simulink model "complete_controller_organized"  (R2023a)
settings: Solver=FixedStepAuto  StartTime=0.0  StopTime=inf  FixedStep=0.01  RelTol=1e-3
model workspace (MAT data in the model file):
  SL_ROS_VariableLengthArrays_MaxSizes.CommonInfo.ArrayTruncateAction = 'EmitWarning'
  SL_ROS_VariableLengthArrays_MaxSizes.MsgTypeMap = containers.Map
  SL_ROS_VariableLengthArrays_MaxSizes.MsgTypeMap.serialization.keys = {'diagnostic_msgs/DiagnosticArray', 'diagnostic_msgs/DiagnosticStatus', 'std_msgs/Float32MultiArray', 'std_msgs/Int32MultiArray'}
  SL_ROS_VariableLengthArrays_MaxSizes.MsgTypeMap.serialization.values{1}.PropertyName = 'status'
  SL_ROS_VariableLengthArrays_MaxSizes.MsgTypeMap.serialization.values{1}.DataType = 'diagnostic_msgs/DiagnosticStatus'
  SL_ROS_VariableLengthArrays_MaxSizes.MsgTypeMap.serialization.values{1}.MaxLength = 2
  SL_ROS_VariableLengthArrays_MaxSizes.MsgTypeMap.serialization.values{2}(1).PropertyName = 'hardware_id'
  SL_ROS_VariableLengthArrays_MaxSizes.MsgTypeMap.serialization.values{2}(1).DataType = 'uint8'
  SL_ROS_VariableLengthArrays_MaxSizes.MsgTypeMap.serialization.values{2}(1).MaxLength = 128
  SL_ROS_VariableLengthArrays_MaxSizes.MsgTypeMap.serialization.values{2}(2).PropertyName = 'message'
  SL_ROS_VariableLengthArrays_MaxSizes.MsgTypeMap.serialization.values{2}(2).DataType = 'uint8'
  SL_ROS_VariableLengthArrays_MaxSizes.MsgTypeMap.serialization.values{2}(2).MaxLength = 128
  SL_ROS_VariableLengthArrays_MaxSizes.MsgTypeMap.serialization.values{2}(3).PropertyName = 'name'
  SL_ROS_VariableLengthArrays_MaxSizes.MsgTypeMap.serialization.values{2}(3).DataType = 'uint8'
  SL_ROS_VariableLengthArrays_MaxSizes.MsgTypeMap.serialization.values{2}(3).MaxLength = 128
  SL_ROS_VariableLengthArrays_MaxSizes.MsgTypeMap.serialization.values{2}(4).PropertyName = 'values'
  SL_ROS_VariableLengthArrays_MaxSizes.MsgTypeMap.serialization.values{2}(4).DataType = 'diagnostic_msgs/KeyValue'
  SL_ROS_VariableLengthArrays_MaxSizes.MsgTypeMap.serialization.values{2}(4).MaxLength = 8
  SL_ROS_VariableLengthArrays_MaxSizes.MsgTypeMap.serialization.values{3}.PropertyName = 'data'
  SL_ROS_VariableLengthArrays_MaxSizes.MsgTypeMap.serialization.values{3}.DataType = 'single'
  SL_ROS_VariableLengthArrays_MaxSizes.MsgTypeMap.serialization.values{3}.MaxLength = 8
  SL_ROS_VariableLengthArrays_MaxSizes.MsgTypeMap.serialization.values{4}.PropertyName = 'data'
  SL_ROS_VariableLengthArrays_MaxSizes.MsgTypeMap.serialization.values{4}.DataType = 'int32'
  SL_ROS_VariableLengthArrays_MaxSizes.MsgTypeMap.serialization.values{4}.MaxLength = 8
  SL_ROS_VariableLengthArrays_MaxSizes.MsgTypeMap.serialization.uniformity = 0
  SL_ROS_VariableLengthArrays_MaxSizes.MsgTypeMap.serialization.keyType = 'char'
  SL_ROS_VariableLengthArrays_MaxSizes.MsgTypeMap.serialization.valueType = 'any'
undefined symbols (not defined in the file): adjusted_FF, angular, Btrigger_boost, DAapply_nudges, DAdesired_pose, DAff_body_force, DAsolver_weights, Djoy_R_X, Dreverse_throttle, Dthrottle, Iangular_mode, Ilinear_mode, linear, reading, standard_variance, status, true_trust
libraries: ros2lib x78
(part 1 of 2)
settings Model: Creator=john  LastModifiedBy=john
settings OptimizationCC: GainParamInheritBuiltInType=on  UseFloatMulNetSlope=on  EnhancedBackFolding=on  PassReuseOutputArgsAs=Individual arguments  ZeroExternalMemoryAtStartup=off  ZeroInternalMemoryAtStartup=off  MaxStackSize=64  OptimizeBlockOrder=speed  DifferentSizesBufferReuse=on  OptimizationCustomize=off  EfficientTunableParamExpr=on
settings DebuggingCC: ParameterTunabilityLossMsg=error  UnderSpecifiedDimensionMsg=warning
settings HardwareCC: ProdBitPerLong=64  ProdHWDeviceType=Intel->x86-64 (Linux 64)
settings SFSimCC: SimUserSources=complete_system/send_thruster_cmd_canbus.c  SimTargetLang=C++
settings RTWCC: Description=Embedded Coder  SystemTargetFile=ert.tlc  HardwareBoard=Robot Operating System 2 (ROS 2)  TLCOptions="-aInlineSetEventsForThisBaseRateFcn=TLC_FALSE -aSuppressMultiTaskScheduler=TLC_FALSE  -aRateBasedStepFcn=0"  TemplateMakefile=ert_default_tmf  Toolchain=Colcon Tools  TargetLang=C++
settings CodeAppCC: ForceParamTrailComments=on  IgnoreCustomStorageClasses=off  OperatorAnnotations=on  SimulinkDataObjDesc=on  SFDataObjDesc=on  InsertBlockDesc=on
settings ERTTargetCC: CodeInterfacePackaging=C++ class  RootIOFormat=Structure reference

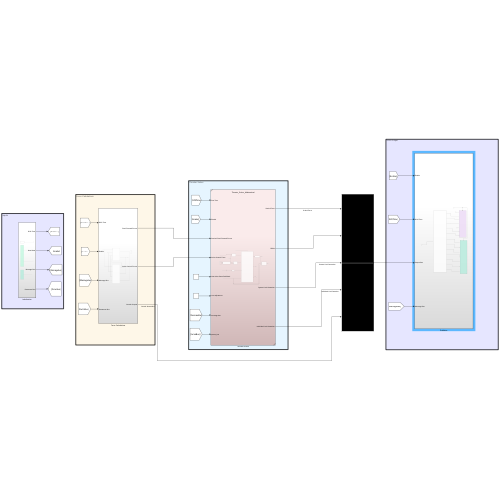
[thumbnail: Simulink's stored preview of the top-level diagram]
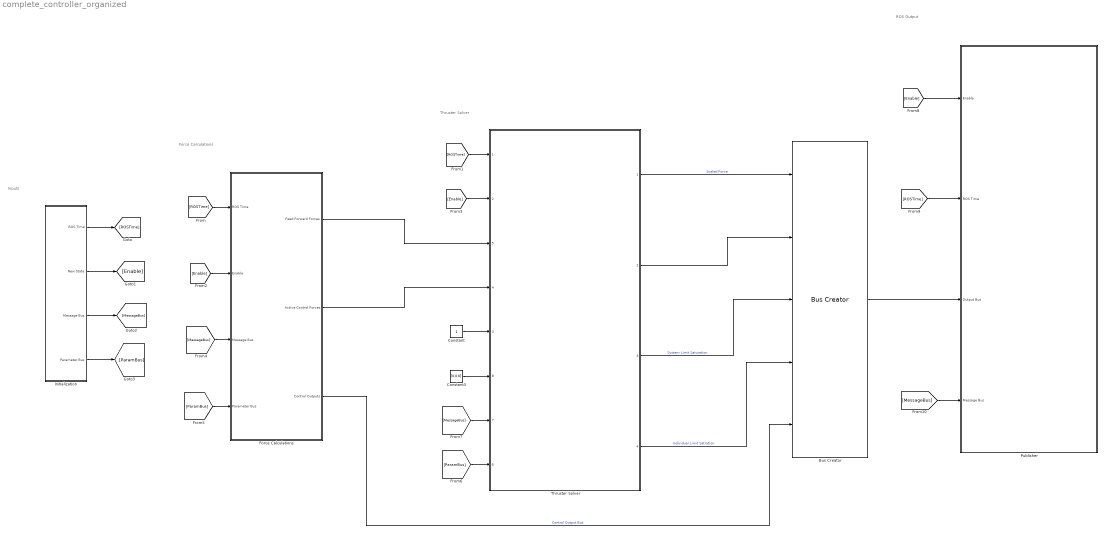
== system complete_controller_organized ==
  note: ROS Output
  note: Thruster Solver
  note: Force Calculations
  note: Inputs
  Bus Creator : BusCreator  Inputs=5
  Constant : Constant
  Constant3 : Constant  Value=[0,0,0]
  Force Calculations : Subsystem
  Initialization : Subsystem
  Publisher : Subsystem
  Thruster Solver : Subsystem  ReferencedSubsystem=Thruster_Solver_Mathmatical
      settings: PortSchema="{\"entries\":[{\"content\":{\"sides\":[{\"content\":{\"connectorIds\":[\"In1\",\"In2\",\"In5\",\"In4\",\"In3\",\"In8\",\"In7\",\"In6\"]},\"type\":\"ConnectorPlacement.EquallySpacedRectSide\",\"uuid\":\"7443c28d-8cee-4065-b63f-8039eaddf426\"},{\"content\":{\"connectorIds\":[\"Out1\",\"Out2\",\"Out3\",\"Out4\"],\"side\":\"RIGHT\"},\"type\":\"ConnectorPlacement.EquallySpacedRectSide\",\"uuid\":\"625b2eba-64d9-4ade-9893-8e78eb613954\"},{\"content\":{\"side\":\"TOP\"},\"type\":\"ConnectorPlacement.EquallySpacedRectSide\",\"uuid\":\"e2df6dfc-d16d-465d-896d-535154799a49\"}]},\"type\":\"ConnectorPlacement.EquallySpacedConnector\",\"uuid\":\"d998c598-ebfe-49fc-a537-223cf8fafed3\"}],\"packageUris\":[\"http://schema.mathworks.com/mf0/Connector/R2020b\"],\"version\":\"1.0\"}"
  wires:
  Force Calculations/1(Feed Forward Forces) -> Thruster Solver/5
  Force Calculations/2(Active Control Forces) -> Thruster Solver/4
  Constant/1 -> Thruster Solver/3
  Constant3/1 -> Thruster Solver/8
  Initialization/1(ROS Time) -> [ROSTime]
  [ROSTime] -> Force Calculations/1(ROS Time)
  [ROSTime] -> Thruster Solver/1
  Initialization/2(New State) -> [Enable]
  [Enable] -> Force Calculations/2(Enable)
  [Enable] -> Thruster Solver/2
  Initialization/3(Message Bus) -> [MessageBus]
  [MessageBus] -> Force Calculations/3(Message Bus)
  Initialization/4(Parameter Bus) -> [ParamBus]
  [ParamBus] -> Force Calculations/4(Parameter Bus)
  [ParamBus] -> Thruster Solver/6
  [MessageBus] -> Thruster Solver/7
  Thruster Solver/1 -> Bus Creator/1  "Scaled Force"
  Thruster Solver/2 -> Bus Creator/2
  Thruster Solver/3 -> Bus Creator/3  "System Limit Saturation"
  Thruster Solver/4 -> Bus Creator/4  "Individual Limit Satration"
  Force Calculations/3(Control Outputs) -> Bus Creator/5  "Control Output Bus"
  Bus Creator/1 -> Publisher/3(Output Bus)
  [Enable] -> Publisher/1(Enable)
  [ROSTime] -> Publisher/2(ROS Time)
  [MessageBus] -> Publisher/4(Message Bus)

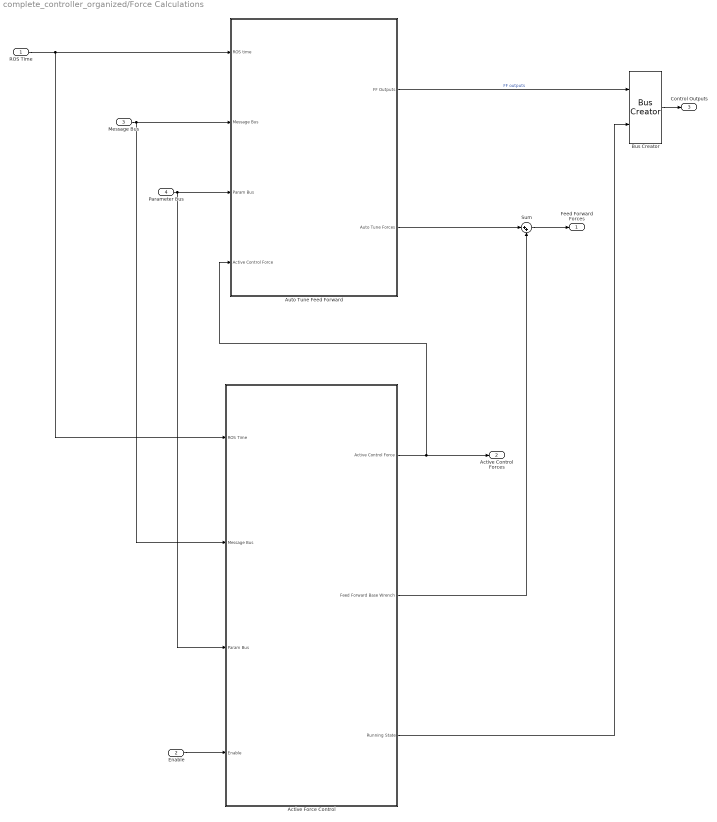
== system complete_controller_organized/Force Calculations ==
  ROS Time : Inport
  Enable : Inport  Port=2
  Message Bus : Inport  Port=3
  Parameter Bus : Inport  Port=4
  Active Force Control : Subsystem
  Auto Tune Feed Forward : Subsystem
  Bus Creator : BusCreator  Inputs=2
  Sum : Sum  Inputs=|++
  Feed Forward Forces : Outport
  Active Control Forces : Outport  Port=2
  Control Outputs : Outport  Port=3
  wires:
  Active Force Control/1(Active Control Force) -> Active Control Forces/1, Auto Tune Feed Forward/4(Active Control Force)
  Sum/1 -> Feed Forward Forces/1
  Auto Tune Feed Forward/2(Auto Tune Forces) -> Sum/1
  Active Force Control/2(Feed Forward Base Wrench) -> Sum/2
  Auto Tune Feed Forward/1(FF Outputs) -> Bus Creator/1  "FF outputs"
  Active Force Control/3(Running State) -> Bus Creator/2
  Bus Creator/1 -> Control Outputs/1
  ROS Time/1 -> Active Force Control/1(ROS Time), Auto Tune Feed Forward/1(ROS time)
  Enable/1 -> Active Force Control/4(Enable)
  Message Bus/1 -> Auto Tune Feed Forward/2(Message Bus), Active Force Control/2(Message Bus)
  Parameter Bus/1 -> Auto Tune Feed Forward/3(Param Bus), Active Force Control/3(Param Bus)

== system complete_controller_organized/Initialization ==
  Current Time : ros2lib/Current Time  OutputFormat=double  SampleTime=-1  ModelName=complete_controller_organized
  Subsystem : Subsystem
  Subsystem1 : Subsystem
  ROS Time : Outport
  New State : Outport  Port=2
  Message Bus : Outport  Port=3
  Parameter Bus : Outport  Port=4
  wires:
  Current Time/1 -> ROS Time/1
  Subsystem1/1(New State) -> New State/1
  Subsystem1/2(Message Bus) -> Message Bus/1
  Subsystem/1(param_bus) -> Parameter Bus/1  "param bus"

== system complete_controller_organized/Publisher ==
  Enable : Inport
  ROS Time : Inport  Port=2
  Output Bus : Inport  Port=3
  Message Bus : Inport  Port=4
  Bus Selector : BusSelector  OutputSignals=RPMs,System Limit Saturation,Individual Limit Satration,Control Output Bus.FF outputs.status,Control Output Bus.FF outputs.reading,Scaled Force,RPMs,Control Output Bus.running_state,Control Output Bus.FF outputs.adjusted_FF,Control Output Bus.FF outputs.reading,Control Output Bus.FF outputs.standard_variance,Control Output Bus.FF outputs.true_trust
  Publish System : Subsystem  ReferencedSubsystem=Publish_Control_System_Out
  Subsystem Reference3 : Subsystem  ReferencedSubsystem=Diagnostic_Reporter
  wires:
  Enable/1 -> Publish System/Enable, Subsystem Reference3/Enable
  Output Bus/1 -> Bus Selector/1
  ROS Time/1 -> Subsystem Reference3/1
  Message Bus/1 -> Subsystem Reference3/5
  Bus Selector/1 -> Subsystem Reference3/2  "<RPMs>"
  Bus Selector/2 -> Subsystem Reference3/3  "<System Limit Saturation>"
  Bus Selector/3 -> Subsystem Reference3/4  "<Individual Limit Satration>"
  Bus Selector/4 -> Subsystem Reference3/6  "<status>"
  Bus Selector/5 -> Subsystem Reference3/7  "<reading>"
  Bus Selector/6 -> Publish System/1  "<Scaled Force>"
  Bus Selector/7 -> Publish System/2  "<RPMs>"
  Bus Selector/8 -> Publish System/3  "<running_state>"
  Bus Selector/9 -> Publish System/4  "<adjusted_FF>"
  Bus Selector/10 -> Publish System/5  "<reading>"
  Bus Selector/11 -> Publish System/6  "<standard_variance>"
  Bus Selector/12 -> Publish System/7  "<true_trust>"

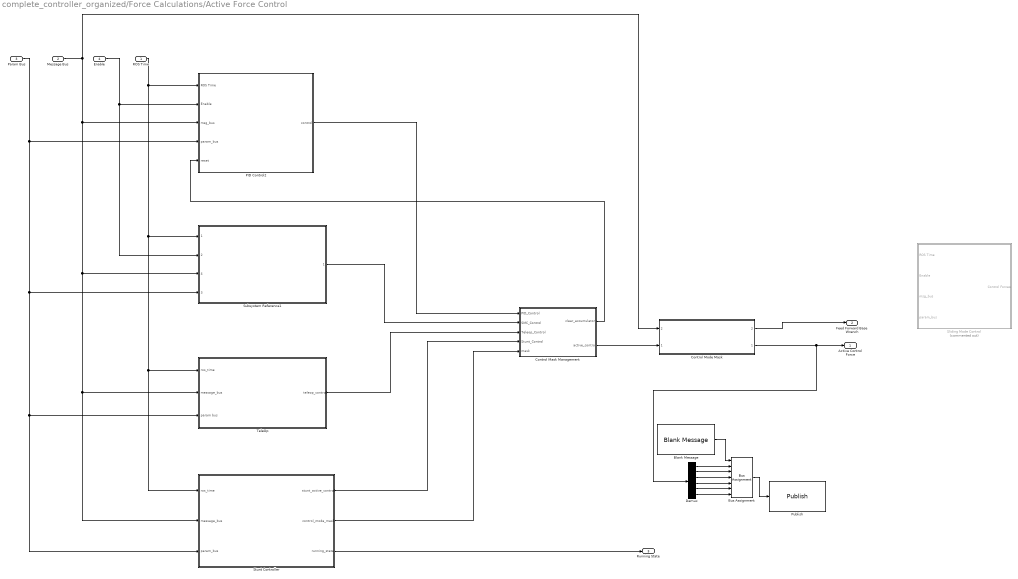
== system complete_controller_organized/Force Calculations/Active Force Control ==
  ROS Time : Inport
  Message Bus : Inport  Port=2
  Param Bus : Inport  Port=3
  Enable : Inport  Port=4
  Blank Message : ros2lib/Blank Message  messageClass=Message  entityType=geometry_msgs/Twist  messageType=geometry_msgs/Twist  SampleTime=inf
  Bus Assignment : BusAssignment  AssignedSignals=linear.x,linear.y,linear.z,angular.x,angular.y,angular.z
  Control Mask Management : Subsystem
  Control Mode Mask : Subsystem  ReferencedSubsystem=Disable_Gains
      settings: PortSchema="{\"entries\":[{\"content\":{\"sides\":[{\"content\":{\"connectorIds\":[\"In2\",\"In1\"]},\"type\":\"ConnectorPlacement.EquallySpacedRectSide\",\"uuid\":\"b7a75f31-ab38-413d-b819-f93313474791\"},{\"content\":{\"connectorIds\":[\"Out2\",\"Out1\"],\"side\":\"RIGHT\"},\"type\":\"ConnectorPlacement.EquallySpacedRectSide\",\"uuid\":\"7159390a-8b2f-48a2-ade8-1d3739d3842f\"},{\"content\":{\"side\":\"TOP\"},\"type\":\"ConnectorPlacement.EquallySpacedRectSide\",\"uuid\":\"3a23d362-7651-42c1-9339-4a667e1f9a44\"}]},\"type\":\"ConnectorPlacement.EquallySpacedConnector\",\"uuid\":\"036ac503-4036-4a11-8f7d-a258a20b039c\"}],\"packageUris\":[\"http://schema.mathworks.com/mf0/Connector/R2020b\"],\"version\":\"1.0\"}"
  Demux : Demux  Outputs=6
  PID Control2 : Subsystem
  Publish : ros2lib/Publish  topicSource=Specify your own  topic=/talos/controller_debug_wrench  messageType=geometry_msgs/Twist  QOSHistory=Keep last  QOSDepth=1  QOSReliability=Reliable  QOSDurability=Volatile
  Sliding Mode Control : Subsystem  Commented=on
  Stunt Controller : Subsystem
  Subsystem Reference1 : Subsystem  ReferencedSubsystem=SMC_mathmatical
      settings: PortSchema="{\"entries\":[{\"content\":{\"sides\":[{\"content\":{\"connectorIds\":[\"In1\",\"In2\",\"In4\",\"In3\"]},\"type\":\"ConnectorPlacement.EquallySpacedRectSide\",\"uuid\":\"d99f1ec8-d0dd-4591-8b28-a91bcf98a65e\"},{\"content\":{\"connectorIds\":[\"Out1\"],\"side\":\"RIGHT\"},\"type\":\"ConnectorPlacement.EquallySpacedRectSide\",\"uuid\":\"f211976d-83c1-4660-96a4-4139d6a3eac5\"},{\"content\":{\"side\":\"TOP\"},\"type\":\"ConnectorPlacement.EquallySpacedRectSide\",\"uuid\":\"9c887152-ce22-4e53-9dff-b8a725742b50\"}]},\"type\":\"ConnectorPlacement.EquallySpacedConnector\",\"uuid\":\"34693693-7ca6-4fc8-a99f-a057e134d206\"}],\"packageUris\":[\"http://schema.mathworks.com/mf0/Connector/R2020b\"],\"version\":\"1.0\"}"
  TeleOp : Subsystem
  Active Control Force : Outport
  Feed Forward Base Wrench : Outport  Port=2
  Running State : Outport  Port=3
  wires:
  ROS Time/1 -> Subsystem Reference1/1, Stunt Controller/1(ros_time), TeleOp/1(ros_time), PID Control2/1(ROS Time)
  Enable/1 -> Subsystem Reference1/2, PID Control2/2(Enable)
  Param Bus/1 -> Stunt Controller/3(param_bus), TeleOp/3(param bus), Subsystem Reference1/3, PID Control2/4(param_bus)
  Stunt Controller/1(stunt_active_control) -> Control Mask Management/4(Stunt_Control)
  Control Mask Management/1(clear_accumulators) -> PID Control2/5(reset)
  PID Control2/1(control) -> Control Mask Management/1(PID_Control)
  Subsystem Reference1/1 -> Control Mask Management/2(SMC_Control)
  TeleOp/1(teleop_control) -> Control Mask Management/3(Teleop_Control)
  Stunt Controller/2(control_mode_mask) -> Control Mask Management/5(mask)
  Stunt Controller/3(running_state) -> Running State/1
  Control Mask Management/2(active_control) -> Control Mode Mask/1
  Control Mode Mask/2 -> Feed Forward Base Wrench/1
  Message Bus/1 -> Stunt Controller/2(message_bus), TeleOp/2(message_bus), Subsystem Reference1/4, PID Control2/3(msg_bus), Control Mode Mask/2
  Demux/1 -> Bus Assignment/2
  Demux/5 -> Bus Assignment/6
  Demux/6 -> Bus Assignment/7
  Demux/3 -> Bus Assignment/4
  Demux/4 -> Bus Assignment/5
  Demux/2 -> Bus Assignment/3
  Blank Message/1 -> Bus Assignment/1
  Bus Assignment/1 -> Publish/1
  Control Mode Mask/1 -> Demux/1, Active Control Force/1

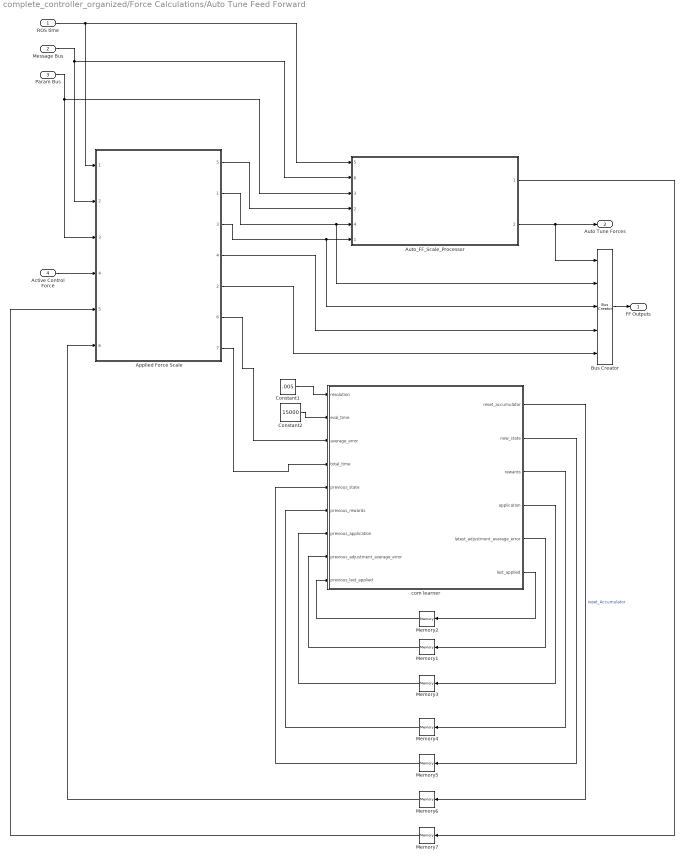
== system complete_controller_organized/Force Calculations/Auto Tune Feed Forward ==
  ROS time : Inport
  Message Bus : Inport  Port=2
  Param Bus : Inport  Port=3
  Active Control Force : Inport  Port=4
  Applied Force Scale : Subsystem  ReferencedSubsystem=AppliedForceScale
      settings: PortSchema="{\"entries\":[{\"content\":{\"sides\":[{\"content\":{\"connectorIds\":[\"In1\",\"In2\",\"In3\",\"In4\",\"In5\",\"In6\"]},\"type\":\"ConnectorPlacement.EquallySpacedRectSide\",\"uuid\":\"e2990854-7279-4b4a-9fa1-c3cb14c90579\"},{\"content\":{\"connectorIds\":[\"Out5\",\"Out1\",\"Out3\",\"Out4\",\"Out2\",\"Out6\",\"Out7\"],\"side\":\"RIGHT\"},\"type\":\"ConnectorPlacement.EquallySpacedRectSide\",\"uuid\":\"eb24cccc-f172-41e0-9329-df49e975e01e\"},{\"content\":{\"side\":\"TOP\"},\"type\":\"ConnectorPlacement.EquallySpacedRectSide\",\"uuid\":\"0d7816fa-ba4f-4eec-b51d-258a96934ff3\"}]},\"type\":\"ConnectorPlacement.EquallySpacedConnector\",\"uuid\":\"161d22c9-7120-4b47-b594-47c184b34751\"}],\"packageUris\":[\"http://schema.mathworks.com/mf0/Connector/R2020b\"],\"version\":\"1.0\"}"
  Auto_FF_Scale_Processor : Subsystem  ReferencedSubsystem=Auto_FF_Scale_Processor
      settings: PortSchema="{\"entries\":[{\"content\":{\"sides\":[{\"content\":{\"connectorIds\":[\"In5\",\"In6\",\"In3\",\"In2\",\"In4\",\"In1\"]},\"type\":\"ConnectorPlacement.EquallySpacedRectSide\",\"uuid\":\"05698164-5f9a-46db-bfeb-335d5ac99d15\"},{\"content\":{\"connectorIds\":[\"Out1\",\"Out2\"],\"side\":\"RIGHT\"},\"type\":\"ConnectorPlacement.EquallySpacedRectSide\",\"uuid\":\"bf55c2a6-1754-464e-aedf-8c76f55d59c0\"},{\"content\":{\"side\":\"TOP\"},\"type\":\"ConnectorPlacement.EquallySpacedRectSide\",\"uuid\":\"da4af13e-a663-4f1d-8ac8-c96129fa845e\"}]},\"type\":\"ConnectorPlacement.EquallySpacedConnector\",\"uuid\":\"5f18ec79-a2ca-4338-bf91-41af61a6ed4d\"}],\"packageUris\":[\"http://schema.mathworks.com/mf0/Connector/R2020b\"],\"version\":\"1.0\"}"
  Bus Creator : BusCreator  Inputs=adjusted_FF,true_trust,reading,standard_variance,status
  Constant1 : Constant  Value=.005
  Constant2 : Constant  Value=15000
  Memory{1..2,5..7} (5 alike) : Memory
  Memory3 : Memory  InitialCondition=[0;0;0]
  Memory4 : Memory  InitialCondition=[0;0;0;0;0;0]
  com learner : MATLAB Function  TreatAsAtomicUnit=on
  FF Outputs : Outport
  Auto Tune Forces : Outport  Port=2
  wires:
  Applied Force Scale/6 -> com learner/3(average_error)
  Applied Force Scale/7 -> com learner/4(total_time)
  Applied Force Scale/3 -> Bus Creator/3, Auto_FF_Scale_Processor/1
  ROS time/1 -> Auto_FF_Scale_Processor/5, Applied Force Scale/1
  Message Bus/1 -> Applied Force Scale/2, Auto_FF_Scale_Processor/6
  Param Bus/1 -> Applied Force Scale/3, Auto_FF_Scale_Processor/3
  Applied Force Scale/5 -> Auto_FF_Scale_Processor/2
  Constant1/1 -> com learner/1(resolution)
  Constant2/1 -> com learner/2(eval_time)
  com learner/6(last_applied) -> Memory2/1
  Memory2/1 -> com learner/9(previous_last_applied)
  com learner/5(latest_adjustment_average_error) -> Memory1/1
  Memory1/1 -> com learner/8(previous_adjustment_average_error)
  com learner/4(application) -> Memory3/1
  Memory3/1 -> com learner/7(previous_application)
  com learner/3(rewards) -> Memory4/1
  Memory4/1 -> com learner/6(previous_rewards)
  com learner/2(new_state) -> Memory5/1
  Memory5/1 -> com learner/5(previous_state)
  com learner/1(reset_accumulator) -> Memory6/1  "reset_Accumulator"
  Active Control Force/1 -> Applied Force Scale/4
  Memory6/1 -> Applied Force Scale/6
  Auto_FF_Scale_Processor/1 -> Memory7/1
  Memory7/1 -> Applied Force Scale/5
  Auto_FF_Scale_Processor/2 -> Bus Creator/1, Auto Tune Forces/1
  Bus Creator/1 -> FF Outputs/1
  Applied Force Scale/1 -> Bus Creator/2, Auto_FF_Scale_Processor/4
  Applied Force Scale/4 -> Bus Creator/4
  Applied Force Scale/2 -> Bus Creator/5

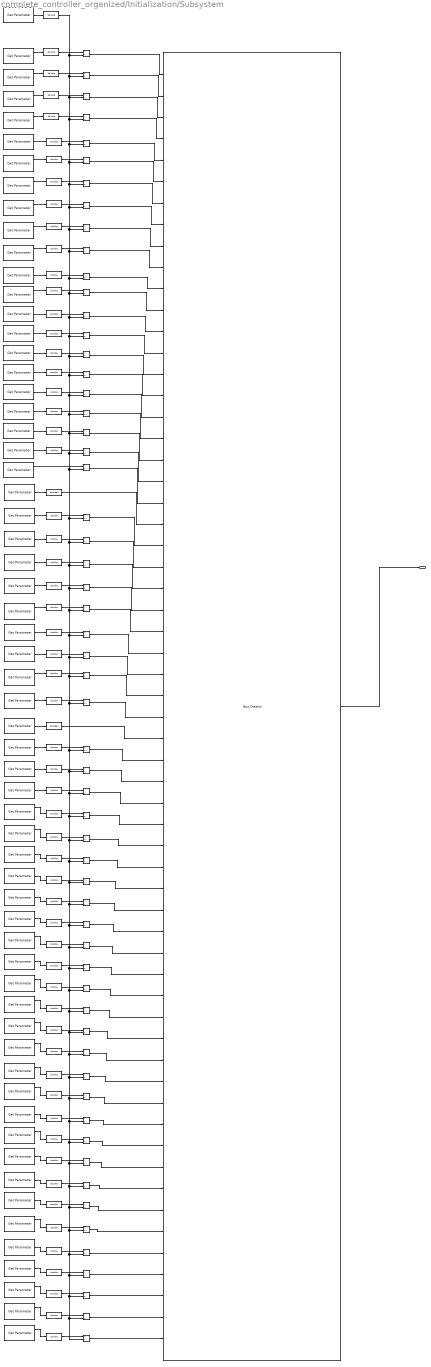
== system complete_controller_organized/Initialization/Subsystem ==
  Active Input Mask : ros2lib/Get Parameter  ParameterName=controller__active_force_mask  ParameterType=int64[]  ParameterMaxArrayLength=6  ParameterInitialValue=[0,0,0,0,0,0]  SampleTime=-1  ModelName=complete_controller_organized  BlockId=ParamGet_complete_controller_organized_59
  Bsnt_safe_mode : DataTypeConversion  OutDataTypeStr=boolean  SaturateOnIntegerOverflow=off  RndMeth=Floor
  Bts_table_mode : DataTypeConversion  OutDataTypeStr=boolean  SaturateOnIntegerOverflow=off  RndMeth=Floor
  DAauto_tune_initial : Product  Inputs=*/
  DAauto_tune_mask : Product  Inputs=*/
  DAd_gains : Product  Inputs=*/
  DAi_gains : Product  Inputs=*/
  DAmax_control : Product  Inputs=*/
  DAnominal_variance : Product  Inputs=*/
  DAp_gains : Product  Inputs=*/
  DAsmc_eta_0 : Product  Inputs=*/
  DAsmc_eta_1 : Product  Inputs=*/
  DAsmc_lamda : Product  Inputs=*/
  DAsmc_max_accelerations : Product  Inputs=*/
  DAsmc_velocity_curve : Product  Inputs=*/
  DAtele_nudge_forces : Product  Inputs=*/
  DAts_rpm_coefficients : Product  Inputs=*/
  DAts_wrenchmat : Product  Inputs=*/
  Data Type Conversion{1,4..14,16..18,20..23} (19 alike) : DataTypeConversion  OutDataTypeStr=double  SaturateOnIntegerOverflow=off  RndMeth=Floor
  Dnominal_time{,1..17} (18 alike) : Product  Inputs=*/
  Dpositional_error_threshold : Product  Inputs=*/
  Dreset_threshold : Product  Inputs=*/
  Dreset_trust_threshold : Product  Inputs=*/
  Dreset_weight_minimum : Product  Inputs=*/
  Dsnt_barrel_roll_duration : Product  Inputs=*/
  Dsnt_barrel_roll_force : Product  Inputs=*/
  Dsnt_summersault_duration : Product  Inputs=*/
  Dsnt_summersault_force : Product  Inputs=*/
  Dtele_accel_force : Product  Inputs=*/
  Dtele_boost_cooldown : Product  Inputs=*/
  Dtele_boost_duration : Product  Inputs=*/
  Dtele_boost_multiplier : Product  Inputs=*/
  Dtele_drag_coefficient : Product  Inputs=*/
  Dtele_reverse_multiplier : Product  Inputs=*/
  Dtele_steering_angle : Product  Inputs=*/
  Dtele_throttle_deadzone : Product  Inputs=*/
  Dtele_width : Product  Inputs=*/
  Dtrust_decay_tau : Product  Inputs=*/
  Dtrust_growth_tau : Product  Inputs=*/
  Dts_disable_weight : Product  Inputs=*/
  Dts_feedback_decay : Product  Inputs=*/
  Dts_individual_thrust_limit : Product  Inputs=*/
  Dts_thrust_limit : Product  Inputs=*/
  Dvelocity_threshold : Product  Inputs=*/
  Eta 0 : ros2lib/Get Parameter  ParameterName=controller__SMC__SMC_params__eta_order_0  ParameterType=int64[]  ParameterMaxArrayLength=6  ParameterInitialValue=0.0  SampleTime=-1  ModelName=complete_controller_organized  BlockId=ParamGet_complete_controller_organized_138
      settings: LibrarySourceBlock=roslib/ROS 2/Get Parameter
  Eta 1 : ros2lib/Get Parameter  ParameterName=controller__SMC__SMC_params__eta_order_1  ParameterType=int64[]  ParameterMaxArrayLength=6  ParameterInitialValue=0.0  SampleTime=-1  ModelName=complete_controller_organized  BlockId=ParamGet_complete_controller_organized_139
      settings: LibrarySourceBlock=roslib/ROS 2/Get Parameter
  Force To Double{,1..38} (39 alike) : DataTypeConversion  OutDataTypeStr=double  SaturateOnIntegerOverflow=off  RndMeth=Floor
  Force To RPM Curve Parameters : ros2lib/Get Parameter  ParameterName=thruster_solver__force_to_rpm_coefficents  ParameterType=int64[]  ParameterMaxArrayLength=8  ParameterInitialValue=[0,0,0,0,0,0,0,0]  SampleTime=-1  ModelName=complete_controller_organized  BlockId=ParamGet_complete_controller_organized_179
      settings: LibrarySourceBlock=roslib/ROS 2/Get Parameter
  Get Parameter : ros2lib/Get Parameter  ParameterName=controller__pid__reset_threshold  ParameterType=int64  ParameterMaxArrayLength=16  ParameterInitialValue=100000  SampleTime=-1  ModelName=complete_controller_organized  BlockId=ParamGet_complete_controller_organized_180
      settings: LibrarySourceBlock=roslib/ROS 2/Get Parameter
  Get Parameter1 : ros2lib/Get Parameter  ParameterName=controller__teleop__width  ParameterType=int64  ParameterMaxArrayLength=16  ParameterInitialValue=900000  SampleTime=-1  ModelName=complete_controller_organized  BlockId=ParamGet_complete_controller_organized_181
  Get Parameter10 : ros2lib/Get Parameter  ParameterName=controller__stunt__summersault_duration  ParameterType=int64  ParameterMaxArrayLength=16  ParameterInitialValue=5000000.0  SampleTime=-1  ModelName=complete_controller_organized  BlockId=ParamGet_complete_controller_organized_182
  Get Parameter11 : ros2lib/Get Parameter  ParameterName=controller__stunt__summersault_force  ParameterType=int64  ParameterMaxArrayLength=16  ParameterInitialValue=20000000  SampleTime=-1  ModelName=complete_controller_organized  BlockId=ParamGet_complete_controller_organized_183
  Get Parameter12 : ros2lib/Get Parameter  ParameterName=controller__stunt__barrel_roll_duration  ParameterType=int64  ParameterMaxArrayLength=16  ParameterInitialValue=4000000.0  SampleTime=-1  ModelName=complete_controller_organized  BlockId=ParamGet_complete_controller_organized_184
  Get Parameter13 : ros2lib/Get Parameter  ParameterName=controller__teleop__boost__cooldown  ParameterType=int64  ParameterMaxArrayLength=16  ParameterInitialValue=10000000  SampleTime=-1  ModelName=complete_controller_organized  BlockId=ParamGet_complete_controller_organized_185
  Get Parameter14 : ros2lib/Get Parameter  ParameterName=controller__teleop__boost__duration  ParameterType=int64  ParameterMaxArrayLength=16  ParameterInitialValue=5000000  SampleTime=-1  ModelName=complete_controller_organized  BlockId=ParamGet_complete_controller_organized_186
  Get Parameter15 : ros2lib/Get Parameter  ParameterName=controller__teleop__boost__multiplier  ParameterType=int64  ParameterMaxArrayLength=16  ParameterInitialValue=1500000  SampleTime=-1  ModelName=complete_controller_organized  BlockId=ParamGet_complete_controller_organized_187
  Get Parameter2 : ros2lib/Get Parameter  ParameterName=controller__teleop__max_steering_angle  ParameterType=int64  ParameterMaxArrayLength=16  ParameterInitialValue=45000000  SampleTime=-1  ModelName=complete_controller_organized  BlockId=ParamGet_complete_controller_organized_188
  Get Parameter3 : ros2lib/Get Parameter  ParameterName=controller__teleop__nudge_forces  ParameterType=int64[]  ParameterMaxArrayLength=6  ParameterInitialValue=[20000000, 20000000, 2000000, 200000, 200000, 2000000]  SampleTime=-1  ModelName=complete_controller_organized  BlockId=ParamGet_complete_controller_organized_189
  Get Parameter4 : ros2lib/Get Parameter  ParameterName=controller__teleop__throttle_deadzone  ParameterType=int64  ParameterMaxArrayLength=16  ParameterInitialValue=50000  SampleTime=-1  ModelName=complete_controller_organized  BlockId=ParamGet_complete_controller_organized_190
  Get Parameter5 : ros2lib/Get Parameter  ParameterName=controller__teleop__reverse_force_multiplier  ParameterType=int64  ParameterMaxArrayLength=16  ParameterInitialValue=400000  SampleTime=-1  ModelName=complete_controller_organized  BlockId=ParamGet_complete_controller_organized_191
  Get Parameter6 : ros2lib/Get Parameter  ParameterName=controller__teleop__drag_coefficient  ParameterType=int64  ParameterMaxArrayLength=16  ParameterInitialValue=420000000  SampleTime=-1  ModelName=complete_controller_organized  BlockId=ParamGet_complete_controller_organized_192
  Get Parameter7 : ros2lib/Get Parameter  ParameterName=controller__teleop__accel_force  ParameterType=int64  ParameterMaxArrayLength=16  ParameterInitialValue=20000000  SampleTime=-1  ModelName=complete_controller_organized  BlockId=ParamGet_complete_controller_organized_193
  Get Parameter8 : ros2lib/Get Parameter  ParameterName=controller__stunt__safe_mode  ParameterType=boolean  ParameterMaxArrayLength=16  ParameterInitialValue=0  SampleTime=-1  ModelName=complete_controller_organized  BlockId=ParamGet_complete_controller_organized_194
  Get Parameter9 : ros2lib/Get Parameter  ParameterName=controller__stunt__barrel_roll_force  ParameterType=int64  ParameterMaxArrayLength=16  ParameterInitialValue=25000000.0  SampleTime=-1  ModelName=complete_controller_organized  BlockId=ParamGet_complete_controller_organized_195
  Get Thruster Wrench Matrix : ros2lib/Get Parameter  ParameterName=talos_wrenchmat  ParameterType=int64[]  ParameterMaxArrayLength=48  ParameterInitialValue=0.0  SampleTime=-1  ModelName=complete_controller_organized  BlockId=ParamGet_complete_controller_organized_196
      settings: LibrarySourceBlock=roslib/ROS 2/Get Parameter
  Iactive_input_mask : Product  Inputs=*/
  Individual Limit : ros2lib/Get Parameter  ParameterName=thruster_solver__individual_thrust_limit  ParameterType=int64  ParameterMaxArrayLength=16  ParameterInitialValue=5.0  SampleTime=-1  ModelName=complete_controller_organized  BlockId=ParamGet_complete_controller_organized_198
      settings: LibrarySourceBlock=roslib/ROS 2/Get Parameter
  Individual Limit1 : ros2lib/Get Parameter  ParameterName=thruster_solver__disable_weight  ParameterType=int64  ParameterMaxArrayLength=16  ParameterInitialValue=10000000  SampleTime=-1  ModelName=complete_controller_organized  BlockId=ParamGet_complete_controller_organized_199
      settings: LibrarySourceBlock=roslib/ROS 2/Get Parameter
  Individual Limit2 : ros2lib/Get Parameter  ParameterName=thruster_solver_table_mode  ParameterType=boolean  ParameterMaxArrayLength=16  ParameterInitialValue=false  SampleTime=-1  ModelName=complete_controller_organized  BlockId=ParamGet_complete_controller_organized_200
      settings: LibrarySourceBlock=roslib/ROS 2/Get Parameter
  Individual Limit3 : ros2lib/Get Parameter  ParameterName=thruster_solver__feedback_decay  ParameterType=int64  ParameterMaxArrayLength=16  ParameterInitialValue=1250000  SampleTime=-1  ModelName=complete_controller_organized  BlockId=ParamGet_complete_controller_organized_201
      settings: LibrarySourceBlock=roslib/ROS 2/Get Parameter
  Param Bus : BusCreator  Inputs=60
  Scaling Factor : ros2lib/Get Parameter  ParameterName=controller__SMC__SMC_params__scaling_factor  ParameterType=int64  ParameterMaxArrayLength=16  ParameterInitialValue=1000000  SampleTime=-1  ModelName=complete_controller_organized  BlockId=ParamGet_complete_controller_organized_203
      settings: LibrarySourceBlock=roslib/ROS 2/Get Parameter
  System Limit : ros2lib/Get Parameter  ParameterName=thruster_solver__system_thrust_limit  ParameterType=int64  ParameterMaxArrayLength=16  ParameterInitialValue=10  SampleTime=-1  ModelName=complete_controller_organized  BlockId=ParamGet_complete_controller_organized_204
      settings: LibrarySourceBlock=roslib/ROS 2/Get Parameter
  convergence threshold1 : ros2lib/Get Parameter  ParameterName=controller__feed_forward__auto_tune__auto_tune_mask  ParameterType=int64[]  ParameterMaxArrayLength=6  ParameterInitialValue=[0;0;0;0;0;0]  SampleTime=-1  ModelName=complete_controller_organized  BlockId=ParamGet_complete_controller_organized_205
      settings: LibrarySourceBlock=roslib/ROS 2/Get Parameter
  convergence threshold10 : ros2lib/Get Parameter  ParameterName=controller__feed_forward__auto_tune__trust_threshold  ParameterType=int64[]  ParameterMaxArrayLength=6  ParameterInitialValue=[970000, 970000, 970000, 970000, 970000, 970000]  SampleTime=-1  ModelName=complete_controller_organized  BlockId=ParamGet_complete_controller_organized_206
      settings: LibrarySourceBlock=roslib/ROS 2/Get Parameter
  convergence threshold11 : ros2lib/Get Parameter  ParameterName=controller__feed_forward__auto_tune__variation_threshold  ParameterType=int64[]  ParameterMaxArrayLength=6  ParameterInitialValue=[1000000, 1000000, 1000000, 1000000, 1000000, 1000000]  SampleTime=-1  ModelName=complete_controller_organized  BlockId=ParamGet_complete_controller_organized_207
      settings: LibrarySourceBlock=roslib/ROS 2/Get Parameter
  convergence threshold12 : ros2lib/Get Parameter  ParameterName=controller__feed_forward__auto_tune__axis_weights  ParameterType=int64[]  ParameterMaxArrayLength=6  ParameterInitialValue=[1000000, 1000000, 1000000, 1000000, 1000000, 1000000]  SampleTime=-1  ModelName=complete_controller_organized  BlockId=ParamGet_complete_controller_organized_208
      settings: LibrarySourceBlock=roslib/ROS 2/Get Parameter
  convergence threshold13 : ros2lib/Get Parameter  ParameterName=controller__feed_forward__auto_tune__variation_der_threshold  ParameterType=int64[]  ParameterMaxArrayLength=6  ParameterInitialValue=[1000000, 1000000, 1000000, 1000000, 1000000, 1000000]  SampleTime=-1  ModelName=complete_controller_organized  BlockId=ParamGet_complete_controller_organized_209
      settings: LibrarySourceBlock=roslib/ROS 2/Get Parameter
  convergence threshold14 : ros2lib/Get Parameter  ParameterName=inertia  ParameterType=int64[]  ParameterMaxArrayLength=3  ParameterInitialValue=[700000,1590000,1650000]  SampleTime=-1  ModelName=complete_controller_organized  BlockId=ParamGet_complete_controller_organized_210
      settings: LibrarySourceBlock=roslib/ROS 2/Get Parameter
  convergence threshold15 : ros2lib/Get Parameter  ParameterName=mass  ParameterType=int64  ParameterMaxArrayLength=6  ParameterInitialValue=32000000  SampleTime=-1  ModelName=complete_controller_organized  BlockId=ParamGet_complete_controller_organized_211
      settings: LibrarySourceBlock=roslib/ROS 2/Get Parameter
  convergence threshold16 : ros2lib/Get Parameter  ParameterName=controller__drag_compensator__apply_mask  ParameterType=int64[]  ParameterMaxArrayLength=36  ParameterInitialValue=zeros(36,1)  SampleTime=-1  ModelName=complete_controller_organized  BlockId=ParamGet_complete_controller_organized_212
      settings: LibrarySourceBlock=roslib/ROS 2/Get Parameter
  convergence threshold17 : ros2lib/Get Parameter  ParameterName=controller__drag_compensator__minimum_samples  ParameterType=int64  ParameterMaxArrayLength=6  ParameterInitialValue=60000000  SampleTime=-1  ModelName=complete_controller_organized  BlockId=ParamGet_complete_controller_organized_213
      settings: LibrarySourceBlock=roslib/ROS 2/Get Parameter
  convergence threshold18 : ros2lib/Get Parameter  ParameterName=controller__drag_compensator__minimum_absolute_velocity  ParameterType=int64  ParameterMaxArrayLength=6  ParameterInitialValue=200000  SampleTime=-1  ModelName=complete_controller_organized  BlockId=ParamGet_complete_controller_organized_214
      settings: LibrarySourceBlock=roslib/ROS 2/Get Parameter
  convergence threshold19 : ros2lib/Get Parameter  ParameterName=controller__drag_compensator__minimum_absolute_positional_error  ParameterType=int64  ParameterMaxArrayLength=3  ParameterInitialValue=200000  SampleTime=-1  ModelName=complete_controller_organized  BlockId=ParamGet_complete_controller_organized_215
      settings: LibrarySourceBlock=roslib/ROS 2/Get Parameter
  convergence threshold2 : ros2lib/Get Parameter  ParameterName=auto_ff__auto_ff  ParameterType=int64[]  ParameterMaxArrayLength=6  ParameterInitialValue=[0;0;0;0;0;0]  SampleTime=-1  ModelName=complete_controller_organized  BlockId=ParamGet_complete_controller_organized_216
      settings: LibrarySourceBlock=roslib/ROS 2/Get Parameter
  convergence threshold20 : ros2lib/Get Parameter  ParameterName=controller__drag_compensator__minimum_average_sampled_velocity  ParameterType=int64[]  ParameterMaxArrayLength=6  ParameterInitialValue=[100000,100000,100000,100000,100000,100000]  SampleTime=-1  ModelName=complete_controller_organized  BlockId=ParamGet_complete_controller_organized_217
      settings: LibrarySourceBlock=roslib/ROS 2/Get Parameter
  convergence threshold21 : ros2lib/Get Parameter  ParameterName=controller__drag_compensator__minimum_R2_coeffiecent  ParameterType=int64  ParameterMaxArrayLength=6  ParameterInitialValue=700000  SampleTime=-1  ModelName=complete_controller_organized  BlockId=ParamGet_complete_controller_organized_218
      settings: LibrarySourceBlock=roslib/ROS 2/Get Parameter
  convergence threshold22 : ros2lib/Get Parameter  ParameterName=controller__drag_compensator__learning_rate  ParameterType=int64  ParameterMaxArrayLength=6  ParameterInitialValue=200000  SampleTime=-1  ModelName=complete_controller_organized  BlockId=ParamGet_complete_controller_organized_219
      settings: LibrarySourceBlock=roslib/ROS 2/Get Parameter
  convergence threshold23 : ros2lib/Get Parameter  ParameterName=controller__drag_compensator__initial_compensation__forward  ParameterType=int64[]  ParameterMaxArrayLength=36  ParameterInitialValue=zeros(36,1)  SampleTime=-1  ModelName=complete_controller_organized  BlockId=ParamGet_complete_controller_organized_220
      settings: LibrarySourceBlock=roslib/ROS 2/Get Parameter
  convergence threshold24 : ros2lib/Get Parameter  ParameterName=controller__autoff__initial_ff  ParameterType=int64[]  ParameterMaxArrayLength=6  ParameterInitialValue=[0,0,0,0,0,0,0]  SampleTime=-1  ModelName=complete_controller_organized  BlockId=ParamGet_complete_controller_organized_221
      settings: LibrarySourceBlock=roslib/ROS 2/Get Parameter
  convergence threshold25 : ros2lib/Get Parameter  ParameterName=controller__drag_compensator__initial_compensation__reverse  ParameterType=int64[]  ParameterMaxArrayLength=36  ParameterInitialValue=zeros(36,1)  SampleTime=-1  ModelName=complete_controller_organized  BlockId=ParamGet_complete_controller_organized_222
      settings: LibrarySourceBlock=roslib/ROS 2/Get Parameter
  convergence threshold3 : ros2lib/Get Parameter  ParameterName=controller__controller_scale__trust_decay_tau  ParameterType=int64  ParameterMaxArrayLength=6  ParameterInitialValue=1000000  SampleTime=-1  ModelName=complete_controller_organized  BlockId=ParamGet_complete_controller_organized_223
      settings: LibrarySourceBlock=roslib/ROS 2/Get Parameter
  convergence threshold4 : ros2lib/Get Parameter  ParameterName=controller__controller_scale__trust_growth_tau  ParameterType=int64  ParameterMaxArrayLength=6  ParameterInitialValue=1000000  SampleTime=-1  ModelName=complete_controller_organized  BlockId=ParamGet_complete_controller_organized_224
      settings: LibrarySourceBlock=roslib/ROS 2/Get Parameter
  convergence threshold5 : ros2lib/Get Parameter  ParameterName=controller__controller_scale__reset_trust_threshold  ParameterType=int64  ParameterMaxArrayLength=200000  ParameterInitialValue=200000  SampleTime=-1  ModelName=complete_controller_organized  BlockId=ParamGet_complete_controller_organized_225
      settings: LibrarySourceBlock=roslib/ROS 2/Get Parameter
  convergence threshold6 : ros2lib/Get Parameter  ParameterName=controller__controller_scale__reset_weight_minimum  ParameterType=int64  ParameterMaxArrayLength=6  ParameterInitialValue=3000000  SampleTime=-1  ModelName=complete_controller_organized  BlockId=ParamGet_complete_controller_organized_226
      settings: LibrarySourceBlock=roslib/ROS 2/Get Parameter
  convergence threshold7 : ros2lib/Get Parameter  ParameterName=controller__controller_scale__nominal_variance  ParameterType=int64[]  ParameterMaxArrayLength=6  ParameterInitialValue=[0;0;0;0;0;0]  SampleTime=-1  ModelName=complete_controller_organized  BlockId=ParamGet_complete_controller_organized_227
      settings: LibrarySourceBlock=roslib/ROS 2/Get Parameter
  convergence threshold8 : ros2lib/Get Parameter  ParameterName=controller__controller_scale__nominal_time  ParameterType=int64  ParameterMaxArrayLength=6  ParameterInitialValue=3000000  SampleTime=-1  ModelName=complete_controller_organized  BlockId=ParamGet_complete_controller_organized_228
      settings: LibrarySourceBlock=roslib/ROS 2/Get Parameter
  convergence threshold9 : ros2lib/Get Parameter  ParameterName=controller__feed_forward__auto_tune__decay_factor  ParameterType=int64[]  ParameterMaxArrayLength=6  ParameterInitialValue=[200000, 200000, 200000, 200000, 200000, 200000]  SampleTime=-1  ModelName=complete_controller_organized  BlockId=ParamGet_complete_controller_organized_229
      settings: LibrarySourceBlock=roslib/ROS 2/Get Parameter
  d Gains : ros2lib/Get Parameter  ParameterName=controller__PID__d_gains  ParameterType=int64[]  ParameterMaxArrayLength=6  ParameterInitialValue=[0,0,0,0,0,0]  SampleTime=-1  ModelName=complete_controller_organized  BlockId=ParamGet_complete_controller_organized_230
      settings: LibrarySourceBlock=roslib/ROS 2/Get Parameter
  error threshold : ros2lib/Get Parameter  ParameterName=controller__feed_forward__auto_tune__positional_error_threshold  ParameterType=int64  ParameterMaxArrayLength=16  ParameterInitialValue=100000  SampleTime=-1  ModelName=complete_controller_organized  BlockId=ParamGet_complete_controller_organized_231
      settings: LibrarySourceBlock=roslib/ROS 2/Get Parameter
  i Gains : ros2lib/Get Parameter  ParameterName=controller__PID__i_gains  ParameterType=int64[]  ParameterMaxArrayLength=6  ParameterInitialValue=[0,0,0,0,0,0]  SampleTime=-1  ModelName=complete_controller_organized  BlockId=ParamGet_complete_controller_organized_232
      settings: LibrarySourceBlock=roslib/ROS 2/Get Parameter
  mass1 : ros2lib/Get Parameter  ParameterName=controller__SMC__SMC_params__velocity_curve_params  ParameterType=int64[]  ParameterMaxArrayLength=12  ParameterInitialValue=[0,0,0,0,0,0,0,0,0,0,0,0]  SampleTime=-1  ModelName=complete_controller_organized  BlockId=ParamGet_complete_controller_organized_233
      settings: LibrarySourceBlock=roslib/ROS 2/Get Parameter
  mass2 : ros2lib/Get Parameter  ParameterName=controller__SMC__max_target_accelerations  ParameterType=int64[]  ParameterMaxArrayLength=6  ParameterInitialValue=[10000,10000,10000,10000,10000,10000]  SampleTime=-1  ModelName=complete_controller_organized  BlockId=ParamGet_complete_controller_organized_234
      settings: LibrarySourceBlock=roslib/ROS 2/Get Parameter
  mass5 : ros2lib/Get Parameter  ParameterName=controller__SMC__SMC_params__lambda  ParameterType=int64[]  ParameterMaxArrayLength=6  ParameterInitialValue=0.0  SampleTime=-1  ModelName=complete_controller_organized  BlockId=ParamGet_complete_controller_organized_235
      settings: LibrarySourceBlock=roslib/ROS 2/Get Parameter
  max_control : ros2lib/Get Parameter  ParameterName=controller__PID__max_control_thresholds  ParameterType=int64[]  ParameterMaxArrayLength=6  ParameterInitialValue=[0,0,0,0,0,0]  SampleTime=-1  ModelName=complete_controller_organized  BlockId=ParamGet_complete_controller_organized_236
      settings: LibrarySourceBlock=roslib/ROS 2/Get Parameter
  p Gains : ros2lib/Get Parameter  ParameterName=controller__PID__p_gains  ParameterType=int64[]  ParameterMaxArrayLength=6  ParameterInitialValue=[0,0,0,0,0,0]  SampleTime=-1  ModelName=complete_controller_organized  BlockId=ParamGet_complete_controller_organized_237
      settings: LibrarySourceBlock=roslib/ROS 2/Get Parameter
  velocity threshold : ros2lib/Get Parameter  ParameterName=controller__feed_forward__auto_tune__velocity_threshold  ParameterType=int64  ParameterMaxArrayLength=16  ParameterInitialValue=100000  SampleTime=-1  ModelName=complete_controller_organized  BlockId=ParamGet_complete_controller_organized_238
      settings: LibrarySourceBlock=roslib/ROS 2/Get Parameter
  param_bus : Outport
  wires:
  Data Type Conversion10/1 -> Dtele_width/1
  Get Parameter4/1 -> Data Type Conversion4/1
  Data Type Conversion22/1 -> Dtele_boost_cooldown/1
  Data Type Conversion20/1 -> Dtele_boost_multiplier/1
  Data Type Conversion11/1 -> Dtele_accel_force/1
  Data Type Conversion23/1 -> DAsmc_max_accelerations/1
  Get Parameter11/1 -> Data Type Conversion16/1
  Get Parameter5/1 -> Data Type Conversion13/1
  Force To RPM Curve Parameters/1 -> Force To Double4/1
  Data Type Conversion13/1 -> Dtele_reverse_multiplier/1
  Get Parameter7/1 -> Data Type Conversion11/1
  Get Parameter1/1 -> Data Type Conversion10/1
  Data Type Conversion21/1 -> Dtele_boost_duration/1
  Get Parameter12/1 -> Data Type Conversion14/1
  Data Type Conversion16/1 -> Dsnt_summersault_force/1
  Scaling Factor/1 -> Force To Double3/1
  Get Parameter6/1 -> Data Type Conversion12/1
  Eta 0/1 -> Data Type Conversion6/1
  Data Type Conversion7/1 -> DAsmc_eta_1/1
  Individual Limit/1 -> Force To Double2/1
  Data Type Conversion8/1 -> DAtele_nudge_forces/1
  Force To Double6/1 -> DAp_gains/1
  p Gains/1 -> Force To Double6/1
  Force To Double5/1 -> Dts_disable_weight/1
  Get Thruster Wrench Matrix/1 -> Force To Double/1
  Get Parameter10/1 -> Data Type Conversion17/1
  Data Type Conversion18/1 -> Dsnt_barrel_roll_force/1
  max_control/1 -> Force To Double11/1
  mass2/1 -> Data Type Conversion23/1
  Get Parameter13/1 -> Data Type Conversion22/1
  Data Type Conversion14/1 -> Dsnt_barrel_roll_duration/1
  Force To Double8/1 -> DAi_gains/1
  Active Input Mask/1 -> Iactive_input_mask/1
  Eta 1/1 -> Data Type Conversion7/1
  Force To Double7/1 -> DAd_gains/1
  Data Type Conversion12/1 -> Dtele_drag_coefficient/1
  d Gains/1 -> Force To Double7/1
  Force To Double4/1 -> DAts_rpm_coefficients/1
  Get Parameter9/1 -> Data Type Conversion18/1
  Get Parameter8/1 -> Bsnt_safe_mode/1
  Individual Limit1/1 -> Force To Double5/1
  Data Type Conversion5/1 -> DAsmc_lamda/1
  mass1/1 -> Data Type Conversion1/1
  Get Parameter/1 -> Force To Double9/1
  Data Type Conversion9/1 -> Dtele_steering_angle/1
  Individual Limit3/1 -> Force To Double10/1
  Get Parameter14/1 -> Data Type Conversion21/1
  mass5/1 -> Data Type Conversion5/1
  System Limit/1 -> Force To Double1/1
  Get Parameter3/1 -> Data Type Conversion8/1
  i Gains/1 -> Force To Double8/1
  Force To Double11/1 -> DAmax_control/1
  Data Type Conversion1/1 -> DAsmc_velocity_curve/1
  Get Parameter15/1 -> Data Type Conversion20/1
  Force To Double1/1 -> Dts_thrust_limit/1
  Data Type Conversion4/1 -> Dtele_throttle_deadzone/1
  Get Parameter2/1 -> Data Type Conversion9/1
  Force To Double9/1 -> Dreset_threshold/1
  Force To Double2/1 -> Dts_individual_thrust_limit/1
  Force To Double10/1 -> Dts_feedback_decay/1
  Data Type Conversion17/1 -> Dsnt_summersault_duration/1
  Data Type Conversion6/1 -> DAsmc_eta_0/1
  Force To Double/1 -> DAts_wrenchmat/1
  Individual Limit2/1 -> Bts_table_mode/1
  Dts_feedback_decay/1 -> Param Bus/33  "Dts_feedback_decay"
  Bts_table_mode/1 -> Param Bus/32  "Bts_table_mode"
  Dts_disable_weight/1 -> Param Bus/31  "Dts_disable_weight"
  DAts_rpm_coefficients/1 -> Param Bus/30  "DAts_rpm_coefficients"
  Dts_individual_thrust_limit/1 -> Param Bus/29  "Dts_individual_thrust_limit"
  Dts_thrust_limit/1 -> Param Bus/28  "Dts_thrust_limit"
  DAts_wrenchmat/1 -> Param Bus/27  "DAts_wrenchmat"
  Dsnt_barrel_roll_duration/1 -> Param Bus/26  "Dsnt_barrel_roll_duration"
  Bsnt_safe_mode/1 -> Param Bus/22  "Bsnt_safe_mode"
  Dsnt_barrel_roll_force/1 -> Param Bus/25  "Dsnt_barrel_roll_force"
  Dsnt_summersault_duration/1 -> Param Bus/24  "Dsnt_summersault_duration"
  Dsnt_summersault_force/1 -> Param Bus/23  "Dsnt_summersault_force"
  Iactive_input_mask/1 -> Param Bus/21  "Iactive_input_mask"
  Dtele_boost_cooldown/1 -> Param Bus/20  "Dtele_boost_cooldown"
  Dtele_boost_duration/1 -> Param Bus/19  "Dtele_boost_duration"
  Dtele_boost_multiplier/1 -> Param Bus/18  "Dtele_boost_multiplier"
  Dtele_reverse_multiplier/1 -> Param Bus/17  "Dtele_reverse_multiplier"
  Dtele_drag_coefficient/1 -> Param Bus/16  "Dtele_drag_coefficient"
  Dtele_accel_force/1 -> Param Bus/15  "Dtele_accel_force"
  Dtele_width/1 -> Param Bus/14  "Dtele_width"
  Dtele_steering_angle/1 -> Param Bus/13  "Dtele_steering_angle"
  DAtele_nudge_forces/1 -> Param Bus/12  "DAtele_nudge_forces"
  Dtele_throttle_deadzone/1 -> Param Bus/11  "Dtele_throttle_deadzone"
  DAsmc_max_accelerations/1 -> Param Bus/10  "DAsmc_max_accelerations"
  DAsmc_velocity_curve/1 -> Param Bus/9  "DAsmc_velocity_curve"
  DAsmc_eta_1/1 -> Param Bus/8  "DAsmc_eta_1"
  DAsmc_eta_0/1 -> Param Bus/7  "DAsmc_eta_0"
  DAsmc_lamda/1 -> Param Bus/6  "DAsmc_lamda"
  Dreset_threshold/1 -> Param Bus/5  "Dreset_threshold"
  DAi_gains/1 -> Param Bus/4  "DAi_gains"
  DAd_gains/1 -> Param Bus/3  "DAd_gains"
  DAp_gains/1 -> Param Bus/2  "DAp_gains"
  DAmax_control/1 -> Param Bus/1  "DAmax_control"
  Param Bus/1 -> param_bus/1
  error threshold/1 -> Force To Double12/1
  velocity threshold/1 -> Force To Double13/1
  Dpositional_error_threshold/1 -> Param Bus/34  "Dpositional_error_threshold"
  Dvelocity_threshold/1 -> Param Bus/35  "Dvelocity_threshold"
  convergence threshold1/1 -> Force To Double19/1
  DAauto_tune_mask/1 -> Param Bus/36  "DAauto_tune_mask"
  Force To Double13/1 -> Dvelocity_threshold/1
  Force To Double12/1 -> Dpositional_error_threshold/1
  Force To Double19/1 -> DAauto_tune_mask/1
  convergence threshold2/1 -> Force To Double20/1
  DAauto_tune_initial/1 -> Param Bus/37  "DAauto_tune_initial"
  Force To Double20/1 -> DAauto_tune_initial/1
  convergence threshold3/1 -> Force To Double21/1
  Dtrust_decay_tau/1 -> Param Bus/38  "Dtrust_decay_tau"
  Force To Double21/1 -> Dtrust_decay_tau/1
  convergence threshold4/1 -> Force To Double22/1
  Dtrust_growth_tau/1 -> Param Bus/39  "Dtrust_growth_tau"
  Force To Double22/1 -> Dtrust_growth_tau/1
  convergence threshold5/1 -> Force To Double23/1
  Dreset_trust_threshold/1 -> Param Bus/40  "Dreset_trust_threshold"
  Force To Double23/1 -> Dreset_trust_threshold/1
  convergence threshold6/1 -> Force To Double24/1
  Dreset_weight_minimum/1 -> Param Bus/41  "Dreset_weight_minimum"
  Force To Double24/1 -> Dreset_weight_minimum/1
  convergence threshold7/1 -> Force To Double25/1
  DAnominal_variance/1 -> Param Bus/42  "DAnominal_variance"
  Force To Double25/1 -> DAnominal_variance/1
  convergence threshold8/1 -> Force To Double26/1
  Dnominal_time/1 -> Param Bus/43  "Dnominal_time"
  Force To Double26/1 -> Dnominal_time/1
  convergence threshold9/1 -> Force To Double27/1
  Force To Double27/1 -> Dnominal_time1/1
  convergence threshold10/1 -> Force To Double28/1
  Force To Double28/1 -> Dnominal_time2/1
  convergence threshold11/1 -> Force To Double29/1
  Force To Double29/1 -> Dnominal_time3/1
  convergence threshold12/1 -> Force To Double30/1
  Force To Double30/1 -> Dnominal_time4/1
  Dnominal_time1/1 -> Param Bus/44  "DAautoff_body_force_decay_percentage"
  Dnominal_time2/1 -> Param Bus/45  "DAautoff_measurement_trust_threshold"
  Dnominal_time3/1 -> Param Bus/46  "DAautoff_standard_variation_threshold"
  Dnominal_time4/1 -> Param Bus/47  "DAautoff_active_force_weights"
  convergence threshold13/1 -> Force To Double14/1
  Force To Double14/1 -> Dnominal_time5/1
  Dnominal_time5/1 -> Param Bus/48  "DAautoff_variation_derivative_threshold"
  Force To Double16/1 -> Dnominal_time6/1
  Dnominal_time6/1 -> Param Bus/49  "DAinterias"
  convergence threshold15/1 -> Force To Double15/1
  Dnominal_time7/1 -> Param Bus/50  "Dmass"
  Force To Double15/1 -> Dnominal_time7/1
  convergence threshold14/1 -> Force To Double16/1
  Dnominal_time13/1 -> Param Bus/55  "DAminimum_drag_update_velocity"
  convergence threshold20/1 -> Force To Double18/1
  Dnominal_time10/1 -> Param Bus/52  "Iminimum_drag_samples"
  Force To Double31/1 -> Dnominal_time12/1
  Dnominal_time11/1 -> Param Bus/53  "Dminimum_drag_sampling_velocity"
  convergence threshold19/1 -> Force To Double31/1
  convergence threshold18/1 -> Force To Double17/1
  Force To Double33/1 -> Dnominal_time10/1
  Dnominal_time12/1 -> Param Bus/54  "Dminimum_drag_positional_error"
  Dnominal_time9/1 -> Param Bus/51  "IAdrag_apply_mask"
  Force To Double17/1 -> Dnominal_time11/1
  convergence threshold17/1 -> Force To Double33/1
  Force To Double32/1 -> Dnominal_time9/1
  convergence threshold16/1 -> Force To Double32/1
  Force To Double18/1 -> Dnominal_time13/1
  convergence threshold21/1 -> Force To Double34/1
  Force To Double34/1 -> Dnominal_time8/1
  Dnominal_time8/1 -> Param Bus/56  "Ddrag_minimum_correspondence_coeffiecent"
  convergence threshold22/1 -> Force To Double35/1
  Dnominal_time14/1 -> Param Bus/57  "Ddrag_learning_rate"
  Force To Double35/1 -> Dnominal_time14/1
  convergence threshold23/1 -> Force To Double36/1
  Dnominal_time15/1 -> Param Bus/58  "DAdrag_init_compensation_forward"
  Force To Double36/1 -> Dnominal_time15/1
  Dnominal_time16/1 -> Param Bus/59  "DAautoff_init_compensation"
  Force To Double37/1 -> Dnominal_time16/1
  convergence threshold24/1 -> Force To Double37/1
  Force To Double3/1 -> Dtele_throttle_deadzone/2, DAtele_nudge_forces/2, Dtele_steering_angle/2, Dtele_width/2, Dtele_accel_force/2, Dtele_drag_coefficient/2, Dtele_boost_multiplier/2, Dtele_boost_duration/2, Dtele_boost_cooldown/2, Dsnt_summersault_force/2, Dsnt_summersault_duration/2, Dsnt_barrel_roll_duration/2, DAts_wrenchmat/2, Dts_thrust_limit/2, Dts_individual_thrust_limit/2, DAts_rpm_coefficients/2, Dvelocity_threshold/2, Dtrust_decay_tau/2, Dtrust_growth_tau/2, Dreset_trust_threshold/2, Dreset_weight_minimum/2, DAnominal_variance/2, Dnominal_time17/2, Dnominal_time16/2, Dnominal_time15/2, Dnominal_time14/2, Dnominal_time8/2, Dnominal_time13/2, Dnominal_time12/2, Dnominal_time11/2, Dnominal_time10/2, Dnominal_time9/2, Dnominal_time7/2, Dnominal_time6/2, Dnominal_time5/2, Dnominal_time4/2, Dnominal_time3/2, Dnominal_time2/2, Dnominal_time1/2, Dnominal_time/2, DAauto_tune_initial/2, DAauto_tune_mask/2, Dpositional_error_threshold/2, Dts_feedback_decay/2, Dts_disable_weight/2, Dsnt_barrel_roll_force/2, Iactive_input_mask/2, Dtele_reverse_multiplier/2, DAsmc_max_accelerations/2, DAsmc_velocity_curve/2, DAsmc_eta_1/2, DAsmc_eta_0/2, DAsmc_lamda/2, Dreset_threshold/2, DAi_gains/2, DAd_gains/2, DAp_gains/2, DAmax_control/2
  Force To Double38/1 -> Dnominal_time17/1
  convergence threshold25/1 -> Force To Double38/1
  Dnominal_time17/1 -> Param Bus/60  "DAdrag_init_compensation_reverse"
